simulink model "Modelo_con_subs_electrico_simulink_PID"  (R2020a)
settings: Solver=ode15s  StartTime=0.0  StopTime=10  FixedStep=0.001  MaxStep=0.001  RelTol=1e-3
undefined symbols (not defined in the file): A, B, ba, Cc, D, f, g, K_motor, K_motor_virtual, ksi, ksia, L, R, R_control, v0, x0
libraries: dspstat3 x1
settings Model: Creator=Noxi-PC  LastModifiedBy=Noxi-PC

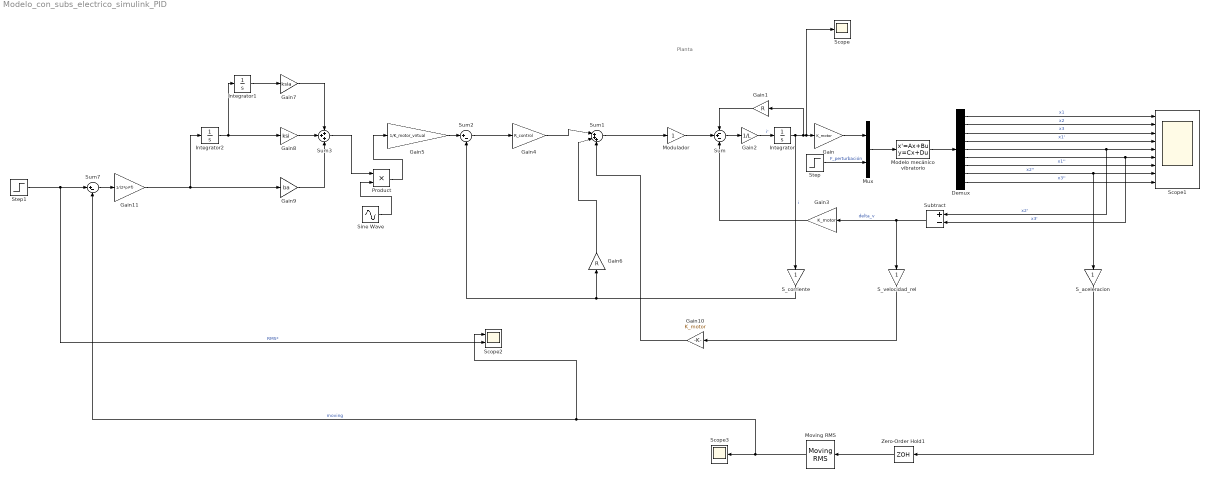
== system Modelo_con_subs_electrico_simulink_PID ==
  note: Planta
  Demux : Demux  Outputs=9
  Gain : Gain  Gain=K_motor
  Gain1 : Gain  Gain=R
  Gain10 : Gain  Gain=K_motor
  Gain11 : Gain  Gain=1/(2*pi*f)
  Gain2 : Gain  Gain=1/L
  Gain3 : Gain  Gain=K_motor
  Gain4 : Gain  Gain=R_control
  Gain5 : Gain  Gain=1/K_motor_virtual
  Gain6 : Gain  Gain=R
  Gain7 : Gain  Gain=ksia
  Gain8 : Gain  Gain=ksi
  Gain9 : Gain  Gain=ba
  Integrator : Integrator
  Integrator1 : Integrator
  Integrator2 : Integrator
  Modelo mecánico vibratorio : StateSpace  A=A  B=B  C=Cc  D=D  InitialCondition=[x0,v0]
  Modulador : Gain
  Moving RMS : dspstat3/Moving RMS  Method=Sliding window  ForgettingFactorPort=off  SpecifyWindowLength=on  WindowLength=Ventana  ForgettingFactor=0.99  SimulateUsing=Code generation
      settings: SourceProductBaseCode=DS
  Mux : Mux  Inputs=2
  Product : Product
  S_aceleracion : Gain
  S_corriente : Gain
  S_velocidad_rel : Gain
  Scope : Scope
  Scope1 : Scope  NumInputPorts=9
  Scope2 : Scope  NumInputPorts=2
  Scope3 : Scope
  Sine Wave : Sin  Frequency=2*pi*f  SampleTime=0
  Step : Step  After=0  SampleTime=0
  Step1 : Step  After=g*2.5/sqrt(2)  SampleTime=0
  Subtract : Sum  Inputs=+-
  Sum : Sum  Inputs=-+-
  Sum1 : Sum  Inputs=|+++
  Sum2 : Sum  Inputs=|+-
  Sum3 : Sum  Inputs=+++
  Sum7 : Sum  Inputs=|+-
  Zero-Order Hold1 : ZeroOrderHold  SampleTime=-1
  wires:
  Modelo mecánico vibratorio/1 -> Demux/1
  Demux/1 -> Scope1/1  "x1"
  Demux/2 -> Scope1/2  "x2"
  Demux/3 -> Scope1/3  "x3"
  Demux/4 -> Scope1/4  "x1'"
  Demux/5 -> Scope1/5, Subtract/1  "x2'"
  Demux/6 -> Scope1/6, Subtract/2  "x3'"
  Demux/7 -> Scope1/7  "x1''"
  Demux/8 -> Scope1/8, S_aceleracion/1  "x2''"
  Demux/9 -> Scope1/9  "x3''"
  Mux/1 -> Modelo mecánico vibratorio/1
  Sum/1 -> Gain2/1
  Integrator/1 -> S_corriente/1, Gain1/1, Scope/1, Gain/1  "i"
  Gain1/1 -> Sum/1
  Gain2/1 -> Integrator/1  "i'"
  Gain/1 -> Mux/1
  Step/1 -> Mux/2  "F_perturbación"
  Gain3/1 -> Sum/3
  Subtract/1 -> S_velocidad_rel/1, Gain3/1  "delta_v"
  Modulador/1 -> Sum/2
  Sum1/1 -> Modulador/1
  Sum2/1 -> Gain4/1
  Gain5/1 -> Sum2/1
  S_corriente/1 -> Gain6/1, Sum2/2
  Gain4/1 -> Sum1/1
  Gain6/1 -> Sum1/2
  Gain8/1 -> Sum3/2
  Gain7/1 -> Sum3/1
  Gain9/1 -> Sum3/3
  Integrator1/1 -> Gain7/1
  Integrator2/1 -> Integrator1/1, Gain8/1
  Gain11/1 -> Gain9/1, Integrator2/1
  S_velocidad_rel/1 -> Gain10/1
  S_aceleracion/1 -> Zero-Order Hold1/1
  Zero-Order Hold1/1 -> Moving RMS/1
  Gain10/1 -> Sum1/3
  Step1/1 -> Scope2/2, Sum7/1  "RMS*"
  Moving RMS/1 -> Scope2/1, Sum7/2, Scope3/1  "moving"
  Sum7/1 -> Gain11/1
  Sine Wave/1 -> Product/2
  Sum3/1 -> Product/1
  Product/1 -> Gain5/1
